simulink model "fake_ros"  (R2020a)
settings: Solver=VariableStepAuto  StartTime=0.0  StopTime=10.0  RelTol=1e-3
undefined symbols (not defined in the file or in its folder): x, y, z
libraries: ros2lib x6, simulink x1
settings Model: Creator=laiy  LastModifiedBy=laiy

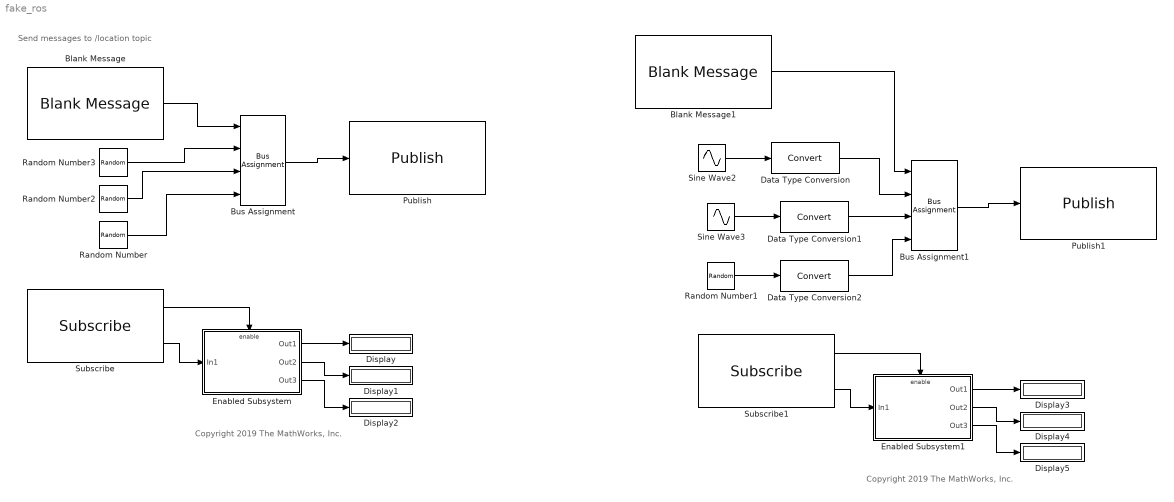
== system fake_ros ==
  note: Copyright 2019 The MathWorks, Inc.
  note: Send messages to /location topic
  note: Copyright 2019 The MathWorks, Inc.
  Blank Message : ros2lib/Blank Message  messageType=geometry_msgs/Point  SampleTime=0.01
      settings: SourceProductBaseCode=RR
  Blank Message1 : ros2lib/Blank Message  messageType=geometry_msgs/Point32  SampleTime=0.01
      settings: SourceProductBaseCode=RR
  Bus Assignment : BusAssignment  AssignedSignals=x,y,z
  Bus Assignment1 : BusAssignment  AssignedSignals=x,y,z
  Data Type Conversion : DataTypeConversion
  Data Type Conversion1 : DataTypeConversion
  Data Type Conversion2 : DataTypeConversion
  Display{,1..5} (6 alike) : Display
  Enabled Subsystem : Subsystem
  Enabled Subsystem1 : Subsystem
  Publish : ros2lib/Publish  topicSource=Specify your own  topic=/velocity  messageType=geometry_msgs/Point  QOSHistory=Keep last  QOSDepth=1  QOSReliability=Reliable  QOSDurability=Volatile
      settings: SourceProductBaseCode=RR
  Publish1 : ros2lib/Publish  topicSource=Specify your own  topic=/bounding_box  messageType=geometry_msgs/Point32  QOSHistory=Keep last  QOSDepth=1  QOSReliability=Reliable  QOSDurability=Volatile
      settings: SourceProductBaseCode=RR
  Random Number{,1..3} (4 alike) : RandomNumber  SampleTime=0.01
  Sine Wave2 : Sin  Phase=-pi/2  SampleTime=0.01  VectorParams1D=off
  Sine Wave3 : Sin  SampleTime=0.01
  Subscribe : ros2lib/Subscribe  topicSource=Specify your own  topic=/velocity  messageType=geometry_msgs/Point  sampleTime=0.01  QOSHistory=Keep last  QOSDepth=1  QOSReliability=Reliable  QOSDurability=Volatile
      settings: SourceProductBaseCode=RR
  Subscribe1 : ros2lib/Subscribe  topicSource=Specify your own  topic=/bounding_box  messageType=geometry_msgs/Point32  sampleTime=0.01  QOSHistory=Keep last  QOSDepth=1  QOSReliability=Reliable  QOSDurability=Volatile
      settings: SourceProductBaseCode=RR
  wires:
  Enabled Subsystem/1(Out1) -> Display/1
  Blank Message/1 -> Bus Assignment/1
  Enabled Subsystem/2(Out2) -> Display1/1
  Subscribe/1 -> Enabled Subsystem/Enable
  Random Number3/1 -> Bus Assignment/2
  Bus Assignment/1 -> Publish/1
  Random Number2/1 -> Bus Assignment/3
  Subscribe/2 -> Enabled Subsystem/1(In1)
  Random Number/1 -> Bus Assignment/4
  Enabled Subsystem/3(Out3) -> Display2/1
  Enabled Subsystem1/3(Out3) -> Display5/1
  Blank Message1/1 -> Bus Assignment1/1
  Subscribe1/2 -> Enabled Subsystem1/1(In1)
  Sine Wave3/1 -> Data Type Conversion1/1
  Subscribe1/1 -> Enabled Subsystem1/Enable
  Enabled Subsystem1/2(Out2) -> Display4/1
  Sine Wave2/1 -> Data Type Conversion/1
  Enabled Subsystem1/1(Out1) -> Display3/1
  Bus Assignment1/1 -> Publish1/1
  Data Type Conversion/1 -> Bus Assignment1/2
  Data Type Conversion1/1 -> Bus Assignment1/3
  Random Number1/1 -> Data Type Conversion2/1
  Data Type Conversion2/1 -> Bus Assignment1/4

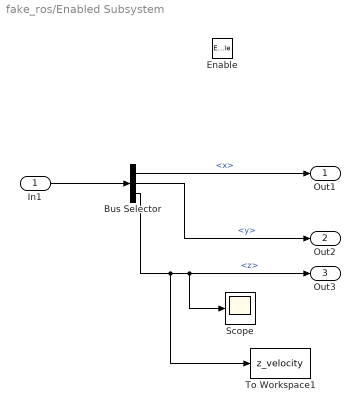
== system fake_ros/Enabled Subsystem ==
  In1 : Inport
  Enable : EnablePort
  Bus Selector : BusSelector  DialogController=Simulink.DDGSource_BusSelector  OutputSignals=x,y,z
  Scope : Scope
  To Workspace1 : ToWorkspace  VariableName=z_velocity  SampleTime=-1
  Out1 : Outport  VectorParamsAs1DForOutWhenUnconnected=off
  Out2 : Outport  Port=2  VectorParamsAs1DForOutWhenUnconnected=off
  Out3 : Outport  Port=3  VectorParamsAs1DForOutWhenUnconnected=off
  wires:
  In1/1 -> Bus Selector/1
  Bus Selector/2 -> Out2/1  "<y>"
  Bus Selector/1 -> Out1/1  "<x>"
  Bus Selector/3 -> To Workspace1/1, Scope/1, Out3/1  "<z>"

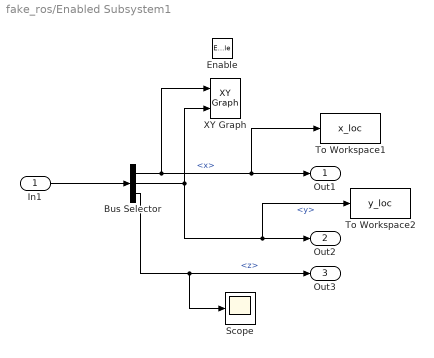
== system fake_ros/Enabled Subsystem1 ==
  In1 : Inport
  Enable : EnablePort
  Bus Selector : BusSelector  DialogController=Simulink.DDGSource_BusSelector  OutputSignals=x,y,z
  Scope : Scope
  To Workspace1 : ToWorkspace  VariableName=x_loc  SampleTime=-1
  To Workspace2 : ToWorkspace  VariableName=y_loc  SampleTime=-1
  XY Graph : simulink/Sinks/XY Graph  xmin=-1  xmax=1  ymin=-1  ymax=1  st=-1
  Out1 : Outport  VectorParamsAs1DForOutWhenUnconnected=off
  Out2 : Outport  Port=2  VectorParamsAs1DForOutWhenUnconnected=off
  Out3 : Outport  Port=3  VectorParamsAs1DForOutWhenUnconnected=off
  wires:
  In1/1 -> Bus Selector/1
  Bus Selector/2 -> To Workspace2/1, Out2/1, XY Graph/2  "<y>"
  Bus Selector/1 -> To Workspace1/1, Out1/1, XY Graph/1  "<x>"
  Bus Selector/3 -> Scope/1, Out3/1  "<z>"
